simulink model "nuclearReactor"  (R2014b)
settings: Solver=ode1  StartTime=0.0  StopTime=100  FixedStep=0.0001  MaxStep=0.0001  RelTol=1e-3
(part 3 of 4)

== system nuclearReactor/Plant6 ==
  control : Inport
  Integrator t0 : DiscreteIntegrator  ExternalReset=either  InitialConditionSource=external  InitialCondition=510  InitialConditionSetting=State (most efficient)  SampleTime=-1
  Integrator t1 : DiscreteIntegrator  ExternalReset=either  InitialConditionSource=external  InitialCondition=510  InitialConditionSetting=State (most efficient)  SampleTime=-1
  Integrator t2 : DiscreteIntegrator  ExternalReset=either  InitialConditionSource=external  InitialCondition=510  InitialConditionSetting=State (most efficient)  SampleTime=-1
  MATLAB Function : MATLAB Function  Priority=1  TreatAsAtomicUnit=on
  MATLAB Function1 : MATLAB Function  Priority=1  TreatAsAtomicUnit=on
  Multiport Switch : MultiPortSwitch  DataPortOrder=Zero-based contiguous
  Scope : Scope  NumInputPorts=8
      settings: TickLabels=on  ShowLegends=on  YMin=0~0~0~10~1~1~0~-1  YMax=40~20~20~30~3~3~1~1
  THR3 : Constant  Value=510
  THR4 : Constant  Value=550
  THR5 : Constant  Value=550
  q : Memory  LinearizeMemory=on
  reset : Memory  LinearizeMemory=on
  x : Outport
  wires:
  Multiport Switch/1 -> Scope/1, MATLAB Function1/1(x), x/1  "x"
  MATLAB Function1/1(x_dot0) -> Integrator t0/1
  THR3/1 -> Integrator t0/3
  THR4/1 -> Integrator t1/3
  THR5/1 -> Integrator t2/3
  Integrator t0/1 -> Scope/2, Multiport Switch/2  "integrator t0"
  Integrator t1/1 -> Scope/3, Multiport Switch/3  "integrator t1"
  Integrator t2/1 -> Scope/4, Multiport Switch/4  "integrator t2"
  MATLAB Function1/2(x_dot1) -> Integrator t1/1
  MATLAB Function1/3(x_dot2) -> Integrator t2/1
  MATLAB Function/1(qNext) -> q/1  "q_before"
  q/1 -> MATLAB Function/1(q), Scope/5, Multiport Switch/1  "q_after"
  control/1 -> Scope/8, MATLAB Function/2(control)
  MATLAB Function/2(reset) -> reset/1
  reset/1 -> Integrator t0/2, Integrator t1/2, Integrator t2/2  "reset_after"

== system nuclearReactor/Plant7 ==
  control : Inport
  Integrator t0 : DiscreteIntegrator  ExternalReset=either  InitialConditionSource=external  InitialCondition=510  InitialConditionSetting=State (most efficient)  SampleTime=-1
  Integrator t1 : DiscreteIntegrator  ExternalReset=either  InitialConditionSource=external  InitialCondition=510  InitialConditionSetting=State (most efficient)  SampleTime=-1
  Integrator t2 : DiscreteIntegrator  ExternalReset=either  InitialConditionSource=external  InitialCondition=510  InitialConditionSetting=State (most efficient)  SampleTime=-1
  MATLAB Function : MATLAB Function  Priority=1  TreatAsAtomicUnit=on
  MATLAB Function1 : MATLAB Function  Priority=1  TreatAsAtomicUnit=on
  Multiport Switch : MultiPortSwitch  DataPortOrder=Zero-based contiguous
  Scope : Scope  NumInputPorts=8
      settings: TickLabels=on  ShowLegends=on  YMin=0~0~0~10~1~1~0~-1  YMax=40~20~20~30~3~3~1~1
  THR3 : Constant  Value=510
  THR4 : Constant  Value=550
  THR5 : Constant  Value=550
  q : Memory  LinearizeMemory=on
  reset : Memory  LinearizeMemory=on
  x : Outport
  wires:
  Multiport Switch/1 -> Scope/1, MATLAB Function1/1(x), x/1  "x"
  MATLAB Function1/1(x_dot0) -> Integrator t0/1
  THR3/1 -> Integrator t0/3
  THR4/1 -> Integrator t1/3
  THR5/1 -> Integrator t2/3
  Integrator t0/1 -> Scope/2, Multiport Switch/2  "integrator t0"
  Integrator t1/1 -> Scope/3, Multiport Switch/3  "integrator t1"
  Integrator t2/1 -> Scope/4, Multiport Switch/4  "integrator t2"
  MATLAB Function1/2(x_dot1) -> Integrator t1/1
  MATLAB Function1/3(x_dot2) -> Integrator t2/1
  MATLAB Function/1(qNext) -> q/1  "q_before"
  q/1 -> MATLAB Function/1(q), Scope/5, Multiport Switch/1  "q_after"
  control/1 -> Scope/8, MATLAB Function/2(control)
  MATLAB Function/2(reset) -> reset/1
  reset/1 -> Integrator t0/2, Integrator t1/2, Integrator t2/2  "reset_after"

== system nuclearReactor/Plant8 ==
  control : Inport
  Integrator t0 : DiscreteIntegrator  ExternalReset=either  InitialConditionSource=external  InitialCondition=510  InitialConditionSetting=State (most efficient)  SampleTime=-1
  Integrator t1 : DiscreteIntegrator  ExternalReset=either  InitialConditionSource=external  InitialCondition=510  InitialConditionSetting=State (most efficient)  SampleTime=-1
  Integrator t2 : DiscreteIntegrator  ExternalReset=either  InitialConditionSource=external  InitialCondition=510  InitialConditionSetting=State (most efficient)  SampleTime=-1
  MATLAB Function : MATLAB Function  Priority=1  TreatAsAtomicUnit=on
  MATLAB Function1 : MATLAB Function  Priority=1  TreatAsAtomicUnit=on
  Multiport Switch : MultiPortSwitch  DataPortOrder=Zero-based contiguous
  Scope : Scope  NumInputPorts=8
      settings: TickLabels=on  ShowLegends=on  YMin=0~0~0~10~1~1~0~-1  YMax=40~20~20~30~3~3~1~1
  THR3 : Constant  Value=510
  THR4 : Constant  Value=550
  THR5 : Constant  Value=550
  q : Memory  LinearizeMemory=on
  reset : Memory  LinearizeMemory=on
  x : Outport
  wires:
  Multiport Switch/1 -> Scope/1, MATLAB Function1/1(x), x/1  "x"
  MATLAB Function1/1(x_dot0) -> Integrator t0/1
  THR3/1 -> Integrator t0/3
  THR4/1 -> Integrator t1/3
  THR5/1 -> Integrator t2/3
  Integrator t0/1 -> Scope/2, Multiport Switch/2  "integrator t0"
  Integrator t1/1 -> Scope/3, Multiport Switch/3  "integrator t1"
  Integrator t2/1 -> Scope/4, Multiport Switch/4  "integrator t2"
  MATLAB Function1/2(x_dot1) -> Integrator t1/1
  MATLAB Function1/3(x_dot2) -> Integrator t2/1
  MATLAB Function/1(qNext) -> q/1  "q_before"
  q/1 -> MATLAB Function/1(q), Scope/5, Multiport Switch/1  "q_after"
  control/1 -> Scope/8, MATLAB Function/2(control)
  MATLAB Function/2(reset) -> reset/1
  reset/1 -> Integrator t0/2, Integrator t1/2, Integrator t2/2  "reset_after"

== system nuclearReactor/Plant9 ==
  control : Inport
  Integrator t0 : DiscreteIntegrator  ExternalReset=either  InitialConditionSource=external  InitialCondition=510  InitialConditionSetting=State (most efficient)  SampleTime=-1
  Integrator t1 : DiscreteIntegrator  ExternalReset=either  InitialConditionSource=external  InitialCondition=510  InitialConditionSetting=State (most efficient)  SampleTime=-1
  Integrator t2 : DiscreteIntegrator  ExternalReset=either  InitialConditionSource=external  InitialCondition=510  InitialConditionSetting=State (most efficient)  SampleTime=-1
  MATLAB Function : MATLAB Function  Priority=1  TreatAsAtomicUnit=on
  MATLAB Function1 : MATLAB Function  Priority=1  TreatAsAtomicUnit=on
  Multiport Switch : MultiPortSwitch  DataPortOrder=Zero-based contiguous
  Scope : Scope  NumInputPorts=8
      settings: TickLabels=on  ShowLegends=on  YMin=0~0~0~10~1~1~0~-1  YMax=40~20~20~30~3~3~1~1
  THR3 : Constant  Value=510
  THR4 : Constant  Value=550
  THR5 : Constant  Value=550
  q : Memory  LinearizeMemory=on
  reset : Memory  LinearizeMemory=on
  x : Outport
  wires:
  Multiport Switch/1 -> Scope/1, MATLAB Function1/1(x), x/1  "x"
  MATLAB Function1/1(x_dot0) -> Integrator t0/1
  THR3/1 -> Integrator t0/3
  THR4/1 -> Integrator t1/3
  THR5/1 -> Integrator t2/3
  Integrator t0/1 -> Scope/2, Multiport Switch/2  "integrator t0"
  Integrator t1/1 -> Scope/3, Multiport Switch/3  "integrator t1"
  Integrator t2/1 -> Scope/4, Multiport Switch/4  "integrator t2"
  MATLAB Function1/2(x_dot1) -> Integrator t1/1
  MATLAB Function1/3(x_dot2) -> Integrator t2/1
  MATLAB Function/1(qNext) -> q/1  "q_before"
  q/1 -> MATLAB Function/1(q), Scope/5, Multiport Switch/1  "q_after"
  control/1 -> Scope/8, MATLAB Function/2(control)
  MATLAB Function/2(reset) -> reset/1
  reset/1 -> Integrator t0/2, Integrator t1/2, Integrator t2/2  "reset_after"

== matlab function nuclearReactor/Plant/MATLAB Function ==
  data: q input; qNext output; control input; reset output


function [qNext,reset]  = phi(q, control)
%#codegen
% control {-1 undefined, 0 add1, 1 remove1, 2 add2, 3 remove2}

undef =0;
add1 = 1;
remove1 =2;
add2 = 3;
remove2 =4;
c=10;

if q==0 
    %When plant is in T0 ("No Rod")
    if control ==add1
        qNext=1;
        reset=1;
    elseif control ==add2
        qNext=2;
        reset=1;
    else
        qNext=0;
        reset=0;
    end;
    
elseif q==1    
    %When plant is in T1 ("Rod One")
    if control ==remove1
        qNext=0;
        reset=1;
    else
        qNext=1;
        reset=0;
    end;

elseif q==2    
    %When plant is in T2 ("Rod Two")
    if control ==remove2
        qNext=0;
        reset=1;
    else
        qNext=2;
        reset=0;
    end;
else
    qNext=-1; %this should never execute
    reset=-1; %this should never execute
end

== matlab function nuclearReactor/Controller/MATLAB Function ==
  data: q input; qNext output; x input; r1 output; r2 output; y1 input; y2 input; control output


function [qNext,r1,r2,control]  = phi(q, x, y1, y2)
%#codegen
% control {-1 undefined, 0 add1, 1 remove1, 2 add2, 3 remove2}

undef =0;
add1 = 1;
remove1 =2;
add2 = 3;
remove2 =4;
c=15;

if q==0 
    %When plant is in T0 ("No Rod")
    if x > 550 && y1 >= c && y2<c
        qNext=1;
        r1=0; r2=0;
        control=add1;
    elseif x>550 && y2>=c
        qNext=2;
        r1=0; r2=0;
        control=add2;
    else
        qNext=0;
        r1=0; r2=0;
        control=undef;
    end;
    
elseif q==1    
    %When plant is in T1 ("Rod One")
    if x <= 510 
        qNext=0;
        r1=1; r2=0;
        control=remove1;
    else
        qNext=1;
        r1=0; r2=0;
        control=undef;
    end;

elseif q==2    
    %When plant is in T2 ("Rod Two")
    if x <= 510 
        qNext=0;
        r1=0; r2=1;
        control=remove2;
    else
        qNext=2;
        r1=0; r2=0;
        control=undef;
    end;
else
    qNext=-1; %this should never execute
    r1=0; r2=0; %this should never execute
    control=-1; %this should never execute
end

== matlab function nuclearReactor/Plant/MATLAB Function1 ==
  data: x input; x_dot0 output; x_dot1 output; x_dot2 output
function [x_dot0, x_dot1, x_dot2] = ODEs(x)
%#codegen
x_dot0=0.1*x-50;
x_dot1=0.1*x-56;
x_dot2=0.1*x-60;

== matlab function nuclearReactor/Controller1/MATLAB Function ==
  data: q input; qNext output; x input; r1 output; r2 output; y1 input; y2 input; control output


function [qNext,r1,r2,control]  = phi(q, x, y1, y2)
%#codegen
% control {-1 undefined, 0 add1, 1 remove1, 2 add2, 3 remove2}

undef =0;
add1 = 1;
remove1 =2;
add2 = 3;
remove2 =4;
c=15;

if q==0 
    %When plant is in T0 ("No Rod")
    if x > 550 && y1 >= c && y2<c
        qNext=1;
        r1=0; r2=0;
        control=add1;
    elseif x>550 && y2>=c
        qNext=2;
        r1=0; r2=0;
        control=add2;
    else
        qNext=0;
        r1=0; r2=0;
        control=undef;
    end;
    
elseif q==1    
    %When plant is in T1 ("Rod One")
    if x <= 510 
        qNext=0;
        r1=1; r2=0;
        control=remove1;
    else
        qNext=1;
        r1=0; r2=0;
        control=undef;
    end;

elseif q==2    
    %When plant is in T2 ("Rod Two")
    if x <= 510 
        qNext=0;
        r1=0; r2=1;
        control=remove2;
    else
        qNext=2;
        r1=0; r2=0;
        control=undef;
    end;
else
    qNext=-1; %this should never execute
    r1=0; r2=0; %this should never execute
    control=-1; %this should never execute
end

== matlab function nuclearReactor/Plant1/MATLAB Function ==
  data: q input; qNext output; control input; reset output


function [qNext,reset]  = phi(q, control)
%#codegen
% control {-1 undefined, 0 add1, 1 remove1, 2 add2, 3 remove2}

undef =0;
add1 = 1;
remove1 =2;
add2 = 3;
remove2 =4;
c=10;

if q==0 
    %When plant is in T0 ("No Rod")
    if control ==add1
        qNext=1;
        reset=1;
    elseif control ==add2
        qNext=2;
        reset=1;
    else
        qNext=0;
        reset=0;
    end;
    
elseif q==1    
    %When plant is in T1 ("Rod One")
    if control ==remove1
        qNext=0;
        reset=1;
    else
        qNext=1;
        reset=0;
    end;

elseif q==2    
    %When plant is in T2 ("Rod Two")
    if control ==remove2
        qNext=0;
        reset=1;
    else
        qNext=2;
        reset=0;
    end;
else
    qNext=-1; %this should never execute
    reset=-1; %this should never execute
end

== matlab function nuclearReactor/Plant1/MATLAB Function1 ==
  data: x input; x_dot0 output; x_dot1 output; x_dot2 output
function [x_dot0, x_dot1, x_dot2] = ODEs(x)
%#codegen
x_dot0=0.1*x-50;
x_dot1=0.1*x-56;
x_dot2=0.1*x-60;

== matlab function nuclearReactor/Controller2/MATLAB Function ==
  data: q input; qNext output; x input; r1 output; r2 output; y1 input; y2 input; control output


function [qNext,r1,r2,control]  = phi(q, x, y1, y2)
%#codegen
% control {-1 undefined, 0 add1, 1 remove1, 2 add2, 3 remove2}

undef =0;
add1 = 1;
remove1 =2;
add2 = 3;
remove2 =4;
c=15;

if q==0 
    %When plant is in T0 ("No Rod")
    if x > 550 && y1 >= c && y2<c
        qNext=1;
        r1=0; r2=0;
        control=add1;
    elseif x>550 && y2>=c
        qNext=2;
        r1=0; r2=0;
        control=add2;
    else
        qNext=0;
        r1=0; r2=0;
        control=undef;
    end;
    
elseif q==1    
    %When plant is in T1 ("Rod One")
    if x <= 510 
        qNext=0;
        r1=1; r2=0;
        control=remove1;
    else
        qNext=1;
        r1=0; r2=0;
        control=undef;
    end;

elseif q==2    
    %When plant is in T2 ("Rod Two")
    if x <= 510 
        qNext=0;
        r1=0; r2=1;
        control=remove2;
    else
        qNext=2;
        r1=0; r2=0;
        control=undef;
    end;
else
    qNext=-1; %this should never execute
    r1=0; r2=0; %this should never execute
    control=-1; %this should never execute
end

== matlab function nuclearReactor/Plant2/MATLAB Function ==
  data: q input; qNext output; control input; reset output


function [qNext,reset]  = phi(q, control)
%#codegen
% control {-1 undefined, 0 add1, 1 remove1, 2 add2, 3 remove2}

undef =0;
add1 = 1;
remove1 =2;
add2 = 3;
remove2 =4;
c=10;

if q==0 
    %When plant is in T0 ("No Rod")
    if control ==add1
        qNext=1;
        reset=1;
    elseif control ==add2
        qNext=2;
        reset=1;
    else
        qNext=0;
        reset=0;
    end;
    
elseif q==1    
    %When plant is in T1 ("Rod One")
    if control ==remove1
        qNext=0;
        reset=1;
    else
        qNext=1;
        reset=0;
    end;

elseif q==2    
    %When plant is in T2 ("Rod Two")
    if control ==remove2
        qNext=0;
        reset=1;
    else
        qNext=2;
        reset=0;
    end;
else
    qNext=-1; %this should never execute
    reset=-1; %this should never execute
end

== matlab function nuclearReactor/Plant2/MATLAB Function1 ==
  data: x input; x_dot0 output; x_dot1 output; x_dot2 output
function [x_dot0, x_dot1, x_dot2] = ODEs(x)
%#codegen
x_dot0=0.1*x-50;
x_dot1=0.1*x-56;
x_dot2=0.1*x-60;

== matlab function nuclearReactor/Controller3/MATLAB Function ==
  data: q input; qNext output; x input; r1 output; r2 output; y1 input; y2 input; control output


function [qNext,r1,r2,control]  = phi(q, x, y1, y2)
%#codegen
% control {-1 undefined, 0 add1, 1 remove1, 2 add2, 3 remove2}

undef =0;
add1 = 1;
remove1 =2;
add2 = 3;
remove2 =4;
c=15;

if q==0 
    %When plant is in T0 ("No Rod")
    if x > 550 && y1 >= c && y2<c
        qNext=1;
        r1=0; r2=0;
        control=add1;
    elseif x>550 && y2>=c
        qNext=2;
        r1=0; r2=0;
        control=add2;
    else
        qNext=0;
        r1=0; r2=0;
        control=undef;
    end;
    
elseif q==1    
    %When plant is in T1 ("Rod One")
    if x <= 510 
        qNext=0;
        r1=1; r2=0;
        control=remove1;
    else
        qNext=1;
        r1=0; r2=0;
        control=undef;
    end;

elseif q==2    
    %When plant is in T2 ("Rod Two")
    if x <= 510 
        qNext=0;
        r1=0; r2=1;
        control=remove2;
    else
        qNext=2;
        r1=0; r2=0;
        control=undef;
    end;
else
    qNext=-1; %this should never execute
    r1=0; r2=0; %this should never execute
    control=-1; %this should never execute
end

== matlab function nuclearReactor/Plant3/MATLAB Function ==
  data: q input; qNext output; control input; reset output


function [qNext,reset]  = phi(q, control)
%#codegen
% control {-1 undefined, 0 add1, 1 remove1, 2 add2, 3 remove2}

undef =0;
add1 = 1;
remove1 =2;
add2 = 3;
remove2 =4;
c=10;

if q==0 
    %When plant is in T0 ("No Rod")
    if control ==add1
        qNext=1;
        reset=1;
    elseif control ==add2
        qNext=2;
        reset=1;
    else
        qNext=0;
        reset=0;
    end;
    
elseif q==1    
    %When plant is in T1 ("Rod One")
    if control ==remove1
        qNext=0;
        reset=1;
    else
        qNext=1;
        reset=0;
    end;

elseif q==2    
    %When plant is in T2 ("Rod Two")
    if control ==remove2
        qNext=0;
        reset=1;
    else
        qNext=2;
        reset=0;
    end;
else
    qNext=-1; %this should never execute
    reset=-1; %this should never execute
end

== matlab function nuclearReactor/Plant3/MATLAB Function1 ==
  data: x input; x_dot0 output; x_dot1 output; x_dot2 output
function [x_dot0, x_dot1, x_dot2] = ODEs(x)
%#codegen
x_dot0=0.1*x-50;
x_dot1=0.1*x-56;
x_dot2=0.1*x-60;

== matlab function nuclearReactor/Controller4/MATLAB Function ==
  data: q input; qNext output; x input; r1 output; r2 output; y1 input; y2 input; control output


function [qNext,r1,r2,control]  = phi(q, x, y1, y2)
%#codegen
% control {-1 undefined, 0 add1, 1 remove1, 2 add2, 3 remove2}

undef =0;
add1 = 1;
remove1 =2;
add2 = 3;
remove2 =4;
c=15;

if q==0 
    %When plant is in T0 ("No Rod")
    if x > 550 && y1 >= c && y2<c
        qNext=1;
        r1=0; r2=0;
        control=add1;
    elseif x>550 && y2>=c
        qNext=2;
        r1=0; r2=0;
        control=add2;
    else
        qNext=0;
        r1=0; r2=0;
        control=undef;
    end;
    
elseif q==1    
    %When plant is in T1 ("Rod One")
    if x <= 510 
        qNext=0;
        r1=1; r2=0;
        control=remove1;
    else
        qNext=1;
        r1=0; r2=0;
        control=undef;
    end;

elseif q==2    
    %When plant is in T2 ("Rod Two")
    if x <= 510 
        qNext=0;
        r1=0; r2=1;
        control=remove2;
    else
        qNext=2;
        r1=0; r2=0;
        control=undef;
    end;
else
    qNext=-1; %this should never execute
    r1=0; r2=0; %this should never execute
    control=-1; %this should never execute
end

== matlab function nuclearReactor/Plant4/MATLAB Function ==
  data: q input; qNext output; control input; reset output


function [qNext,reset]  = phi(q, control)
%#codegen
% control {-1 undefined, 0 add1, 1 remove1, 2 add2, 3 remove2}

undef =0;
add1 = 1;
remove1 =2;
add2 = 3;
remove2 =4;
c=10;

if q==0 
    %When plant is in T0 ("No Rod")
    if control ==add1
        qNext=1;
        reset=1;
    elseif control ==add2
        qNext=2;
        reset=1;
    else
        qNext=0;
        reset=0;
    end;
    
elseif q==1    
    %When plant is in T1 ("Rod One")
    if control ==remove1
        qNext=0;
        reset=1;
    else
        qNext=1;
        reset=0;
    end;

elseif q==2    
    %When plant is in T2 ("Rod Two")
    if control ==remove2
        qNext=0;
        reset=1;
    else
        qNext=2;
        reset=0;
    end;
else
    qNext=-1; %this should never execute
    reset=-1; %this should never execute
end

== matlab function nuclearReactor/Plant4/MATLAB Function1 ==
  data: x input; x_dot0 output; x_dot1 output; x_dot2 output
function [x_dot0, x_dot1, x_dot2] = ODEs(x)
%#codegen
x_dot0=0.1*x-50;
x_dot1=0.1*x-56;
x_dot2=0.1*x-60;

== matlab function nuclearReactor/Controller5/MATLAB Function ==
  data: q input; qNext output; x input; r1 output; r2 output; y1 input; y2 input; control output


function [qNext,r1,r2,control]  = phi(q, x, y1, y2)
%#codegen
% control {-1 undefined, 0 add1, 1 remove1, 2 add2, 3 remove2}

undef =0;
add1 = 1;
remove1 =2;
add2 = 3;
remove2 =4;
c=15;

if q==0 
    %When plant is in T0 ("No Rod")
    if x > 550 && y1 >= c && y2<c
        qNext=1;
        r1=0; r2=0;
        control=add1;
    elseif x>550 && y2>=c
        qNext=2;
        r1=0; r2=0;
        control=add2;
    else
        qNext=0;
        r1=0; r2=0;
        control=undef;
    end;
    
elseif q==1    
    %When plant is in T1 ("Rod One")
    if x <= 510 
        qNext=0;
        r1=1; r2=0;
        control=remove1;
    else
        qNext=1;
        r1=0; r2=0;
        control=undef;
    end;

elseif q==2    
    %When plant is in T2 ("Rod Two")
    if x <= 510 
        qNext=0;
        r1=0; r2=1;
        control=remove2;
    else
        qNext=2;
        r1=0; r2=0;
        control=undef;
    end;
else
    qNext=-1; %this should never execute
    r1=0; r2=0; %this should never execute
    control=-1; %this should never execute
end

== matlab function nuclearReactor/Plant5/MATLAB Function ==
  data: q input; qNext output; control input; reset output


function [qNext,reset]  = phi(q, control)
%#codegen
% control {-1 undefined, 0 add1, 1 remove1, 2 add2, 3 remove2}

undef =0;
add1 = 1;
remove1 =2;
add2 = 3;
remove2 =4;
c=10;

if q==0 
    %When plant is in T0 ("No Rod")
    if control ==add1
        qNext=1;
        reset=1;
    elseif control ==add2
        qNext=2;
        reset=1;
    else
        qNext=0;
        reset=0;
    end;
    
elseif q==1    
    %When plant is in T1 ("Rod One")
    if control ==remove1
        qNext=0;
        reset=1;
    else
        qNext=1;
        reset=0;
    end;

elseif q==2    
    %When plant is in T2 ("Rod Two")
    if control ==remove2
        qNext=0;
        reset=1;
    else
        qNext=2;
        reset=0;
    end;
else
    qNext=-1; %this should never execute
    reset=-1; %this should never execute
end

== matlab function nuclearReactor/Plant5/MATLAB Function1 ==
  data: x input; x_dot0 output; x_dot1 output; x_dot2 output
function [x_dot0, x_dot1, x_dot2] = ODEs(x)
%#codegen
x_dot0=0.1*x-50;
x_dot1=0.1*x-56;
x_dot2=0.1*x-60;

== matlab function nuclearReactor/Controller6/MATLAB Function ==
  data: q input; qNext output; x input; r1 output; r2 output; y1 input; y2 input; control output


function [qNext,r1,r2,control]  = phi(q, x, y1, y2)
%#codegen
% control {-1 undefined, 0 add1, 1 remove1, 2 add2, 3 remove2}

undef =0;
add1 = 1;
remove1 =2;
add2 = 3;
remove2 =4;
c=15;

if q==0 
    %When plant is in T0 ("No Rod")
    if x > 550 && y1 >= c && y2<c
        qNext=1;
        r1=0; r2=0;
        control=add1;
    elseif x>550 && y2>=c
        qNext=2;
        r1=0; r2=0;
        control=add2;
    else
        qNext=0;
        r1=0; r2=0;
        control=undef;
    end;
    
elseif q==1    
    %When plant is in T1 ("Rod One")
    if x <= 510 
        qNext=0;
        r1=1; r2=0;
        control=remove1;
    else
        qNext=1;
        r1=0; r2=0;
        control=undef;
    end;

elseif q==2    
    %When plant is in T2 ("Rod Two")
    if x <= 510 
        qNext=0;
        r1=0; r2=1;
        control=remove2;
    else
        qNext=2;
        r1=0; r2=0;
        control=undef;
    end;
else
    qNext=-1; %this should never execute
    r1=0; r2=0; %this should never execute
    control=-1; %this should never execute
end

== matlab function nuclearReactor/Plant6/MATLAB Function ==
  data: q input; qNext output; control input; reset output


function [qNext,reset]  = phi(q, control)
%#codegen
% control {-1 undefined, 0 add1, 1 remove1, 2 add2, 3 remove2}

undef =0;
add1 = 1;
remove1 =2;
add2 = 3;
remove2 =4;
c=10;

if q==0 
    %When plant is in T0 ("No Rod")
    if control ==add1
        qNext=1;
        reset=1;
    elseif control ==add2
        qNext=2;
        reset=1;
    else
        qNext=0;
        reset=0;
    end;
    
elseif q==1    
    %When plant is in T1 ("Rod One")
    if control ==remove1
        qNext=0;
        reset=1;
    else
        qNext=1;
        reset=0;
    end;

elseif q==2    
    %When plant is in T2 ("Rod Two")
    if control ==remove2
        qNext=0;
        reset=1;
    else
        qNext=2;
        reset=0;
    end;
else
    qNext=-1; %this should never execute
    reset=-1; %this should never execute
end

== matlab function nuclearReactor/Plant6/MATLAB Function1 ==
  data: x input; x_dot0 output; x_dot1 output; x_dot2 output
function [x_dot0, x_dot1, x_dot2] = ODEs(x)
%#codegen
x_dot0=0.1*x-50;
x_dot1=0.1*x-56;
x_dot2=0.1*x-60;

== matlab function nuclearReactor/Controller7/MATLAB Function ==
  data: q input; qNext output; x input; r1 output; r2 output; y1 input; y2 input; control output


function [qNext,r1,r2,control]  = phi(q, x, y1, y2)
%#codegen
% control {-1 undefined, 0 add1, 1 remove1, 2 add2, 3 remove2}

undef =0;
add1 = 1;
remove1 =2;
add2 = 3;
remove2 =4;
c=15;

if q==0 
    %When plant is in T0 ("No Rod")
    if x > 550 && y1 >= c && y2<c
        qNext=1;
        r1=0; r2=0;
        control=add1;
    elseif x>550 && y2>=c
        qNext=2;
        r1=0; r2=0;
        control=add2;
    else
        qNext=0;
        r1=0; r2=0;
        control=undef;
    end;
    
elseif q==1    
    %When plant is in T1 ("Rod One")
    if x <= 510 
        qNext=0;
        r1=1; r2=0;
        control=remove1;
    else
        qNext=1;
        r1=0; r2=0;
        control=undef;
    end;

elseif q==2    
    %When plant is in T2 ("Rod Two")
    if x <= 510 
        qNext=0;
        r1=0; r2=1;
        control=remove2;
    else
        qNext=2;
        r1=0; r2=0;
        control=undef;
    end;
else
    qNext=-1; %this should never execute
    r1=0; r2=0; %this should never execute
    control=-1; %this should never execute
end

== matlab function nuclearReactor/Plant7/MATLAB Function ==
  data: q input; qNext output; control input; reset output


function [qNext,reset]  = phi(q, control)
%#codegen
% control {-1 undefined, 0 add1, 1 remove1, 2 add2, 3 remove2}

undef =0;
add1 = 1;
remove1 =2;
add2 = 3;
remove2 =4;
c=10;

if q==0 
    %When plant is in T0 ("No Rod")
    if control ==add1
        qNext=1;
        reset=1;
    elseif control ==add2
        qNext=2;
        reset=1;
    else
        qNext=0;
        reset=0;
    end;
    
elseif q==1    
    %When plant is in T1 ("Rod One")
    if control ==remove1
        qNext=0;
        reset=1;
    else
        qNext=1;
        reset=0;
    end;

elseif q==2    
    %When plant is in T2 ("Rod Two")
    if control ==remove2
        qNext=0;
        reset=1;
    else
        qNext=2;
        reset=0;
    end;
else
    qNext=-1; %this should never execute
    reset=-1; %this should never execute
end

== matlab function nuclearReactor/Plant7/MATLAB Function1 ==
  data: x input; x_dot0 output; x_dot1 output; x_dot2 output
function [x_dot0, x_dot1, x_dot2] = ODEs(x)
%#codegen
x_dot0=0.1*x-50;
x_dot1=0.1*x-56;
x_dot2=0.1*x-60;

== matlab function nuclearReactor/Controller8/MATLAB Function ==
  data: q input; qNext output; x input; r1 output; r2 output; y1 input; y2 input; control output


function [qNext,r1,r2,control]  = phi(q, x, y1, y2)
%#codegen
% control {-1 undefined, 0 add1, 1 remove1, 2 add2, 3 remove2}

undef =0;
add1 = 1;
remove1 =2;
add2 = 3;
remove2 =4;
c=15;

if q==0 
    %When plant is in T0 ("No Rod")
    if x > 550 && y1 >= c && y2<c
        qNext=1;
        r1=0; r2=0;
        control=add1;
    elseif x>550 && y2>=c
        qNext=2;
        r1=0; r2=0;
        control=add2;
    else
        qNext=0;
        r1=0; r2=0;
        control=undef;
    end;
    
elseif q==1    
    %When plant is in T1 ("Rod One")
    if x <= 510 
        qNext=0;
        r1=1; r2=0;
        control=remove1;
    else
        qNext=1;
        r1=0; r2=0;
        control=undef;
    end;

elseif q==2    
    %When plant is in T2 ("Rod Two")
    if x <= 510 
        qNext=0;
        r1=0; r2=1;
        control=remove2;
    else
        qNext=2;
        r1=0; r2=0;
        control=undef;
    end;
else
    qNext=-1; %this should never execute
    r1=0; r2=0; %this should never execute
    control=-1; %this should never execute
end

== matlab function nuclearReactor/Plant8/MATLAB Function ==
  data: q input; qNext output; control input; reset output


function [qNext,reset]  = phi(q, control)
%#codegen
% control {-1 undefined, 0 add1, 1 remove1, 2 add2, 3 remove2}

undef =0;
add1 = 1;
remove1 =2;
add2 = 3;
remove2 =4;
c=10;

if q==0 
    %When plant is in T0 ("No Rod")
    if control ==add1
        qNext=1;
        reset=1;
    elseif control ==add2
        qNext=2;
        reset=1;
    else
        qNext=0;
        reset=0;
    end;
    
elseif q==1    
    %When plant is in T1 ("Rod One")
    if control ==remove1
        qNext=0;
        reset=1;
    else
        qNext=1;
        reset=0;
    end;

elseif q==2    
    %When plant is in T2 ("Rod Two")
    if control ==remove2
        qNext=0;
        reset=1;
    else
        qNext=2;
        reset=0;
    end;
else
    qNext=-1; %this should never execute
    reset=-1; %this should never execute
end

== matlab function nuclearReactor/Plant8/MATLAB Function1 ==
  data: x input; x_dot0 output; x_dot1 output; x_dot2 output
function [x_dot0, x_dot1, x_dot2] = ODEs(x)
%#codegen
x_dot0=0.1*x-50;
x_dot1=0.1*x-56;
x_dot2=0.1*x-60;

== matlab function nuclearReactor/Controller9/MATLAB Function ==
  data: q input; qNext output; x input; r1 output; r2 output; y1 input; y2 input; control output


function [qNext,r1,r2,control]  = phi(q, x, y1, y2)
%#codegen
% control {-1 undefined, 0 add1, 1 remove1, 2 add2, 3 remove2}

undef =0;
add1 = 1;
remove1 =2;
add2 = 3;
remove2 =4;
c=15;

if q==0 
    %When plant is in T0 ("No Rod")
    if x > 550 && y1 >= c && y2<c
        qNext=1;
        r1=0; r2=0;
        control=add1;
    elseif x>550 && y2>=c
        qNext=2;
        r1=0; r2=0;
        control=add2;
    else
        qNext=0;
        r1=0; r2=0;
        control=undef;
    end;
    
elseif q==1    
    %When plant is in T1 ("Rod One")
    if x <= 510 
        qNext=0;
        r1=1; r2=0;
        control=remove1;
    else
        qNext=1;
        r1=0; r2=0;
        control=undef;
    end;

elseif q==2    
    %When plant is in T2 ("Rod Two")
    if x <= 510 
        qNext=0;
        r1=0; r2=1;
        control=remove2;
    else
        qNext=2;
        r1=0; r2=0;
        control=undef;
    end;
else
    qNext=-1; %this should never execute
    r1=0; r2=0; %this should never execute
    control=-1; %this should never execute
end

== matlab function nuclearReactor/Plant9/MATLAB Function ==
  data: q input; qNext output; control input; reset output


function [qNext,reset]  = phi(q, control)
%#codegen
% control {-1 undefined, 0 add1, 1 remove1, 2 add2, 3 remove2}

undef =0;
add1 = 1;
remove1 =2;
add2 = 3;
remove2 =4;
c=10;

if q==0 
    %When plant is in T0 ("No Rod")
    if control ==add1
        qNext=1;
        reset=1;
    elseif control ==add2
        qNext=2;
        reset=1;
    else
        qNext=0;
        reset=0;
    end;
    
elseif q==1    
    %When plant is in T1 ("Rod One")
    if control ==remove1
        qNext=0;
        reset=1;
    else
        qNext=1;
        reset=0;
    end;

elseif q==2    
    %When plant is in T2 ("Rod Two")
    if control ==remove2
        qNext=0;
        reset=1;
    else
        qNext=2;
        reset=0;
    end;
else
    qNext=-1; %this should never execute
    reset=-1; %this should never execute
end

== matlab function nuclearReactor/Plant9/MATLAB Function1 ==
  data: x input; x_dot0 output; x_dot1 output; x_dot2 output
function [x_dot0, x_dot1, x_dot2] = ODEs(x)
%#codegen
x_dot0=0.1*x-50;
x_dot1=0.1*x-56;
x_dot2=0.1*x-60;

== matlab function nuclearReactor/Controller10/MATLAB Function ==
  data: q input; qNext output; x input; r1 output; r2 output; y1 input; y2 input; control output


function [qNext,r1,r2,control]  = phi(q, x, y1, y2)
%#codegen
% control {-1 undefined, 0 add1, 1 remove1, 2 add2, 3 remove2}

undef =0;
add1 = 1;
remove1 =2;
add2 = 3;
remove2 =4;
c=15;

if q==0 
    %When plant is in T0 ("No Rod")
    if x > 550 && y1 >= c && y2<c
        qNext=1;
        r1=0; r2=0;
        control=add1;
    elseif x>550 && y2>=c
        qNext=2;
        r1=0; r2=0;
        control=add2;
    else
        qNext=0;
        r1=0; r2=0;
        control=undef;
    end;
    
elseif q==1    
    %When plant is in T1 ("Rod One")
    if x <= 510 
        qNext=0;
        r1=1; r2=0;
        control=remove1;
    else
        qNext=1;
        r1=0; r2=0;
        control=undef;
    end;

elseif q==2    
    %When plant is in T2 ("Rod Two")
    if x <= 510 
        qNext=0;
        r1=0; r2=1;
        control=remove2;
    else
        qNext=2;
        r1=0; r2=0;
        control=undef;
    end;
else
    qNext=-1; %this should never execute
    r1=0; r2=0; %this should never execute
    control=-1; %this should never execute
end

== matlab function nuclearReactor/Plant10/MATLAB Function ==
  data: q input; qNext output; control input; reset output


function [qNext,reset]  = phi(q, control)
%#codegen
% control {-1 undefined, 0 add1, 1 remove1, 2 add2, 3 remove2}

undef =0;
add1 = 1;
remove1 =2;
add2 = 3;
remove2 =4;
c=10;

if q==0 
    %When plant is in T0 ("No Rod")
    if control ==add1
        qNext=1;
        reset=1;
    elseif control ==add2
        qNext=2;
        reset=1;
    else
        qNext=0;
        reset=0;
    end;
    
elseif q==1    
    %When plant is in T1 ("Rod One")
    if control ==remove1
        qNext=0;
        reset=1;
    else
        qNext=1;
        reset=0;
    end;

elseif q==2    
    %When plant is in T2 ("Rod Two")
    if control ==remove2
        qNext=0;
        reset=1;
    else
        qNext=2;
        reset=0;
    end;
else
    qNext=-1; %this should never execute
    reset=-1; %this should never execute
end

== matlab function nuclearReactor/Plant10/MATLAB Function1 ==
  data: x input; x_dot0 output; x_dot1 output; x_dot2 output
function [x_dot0, x_dot1, x_dot2] = ODEs(x)
%#codegen
x_dot0=0.1*x-50;
x_dot1=0.1*x-56;
x_dot2=0.1*x-60;

== matlab function nuclearReactor/Controller11/MATLAB Function ==
  data: q input; qNext output; x input; r1 output; r2 output; y1 input; y2 input; control output


function [qNext,r1,r2,control]  = phi(q, x, y1, y2)
%#codegen
% control {-1 undefined, 0 add1, 1 remove1, 2 add2, 3 remove2}

undef =0;
add1 = 1;
remove1 =2;
add2 = 3;
remove2 =4;
c=15;

if q==0 
    %When plant is in T0 ("No Rod")
    if x > 550 && y1 >= c && y2<c
        qNext=1;
        r1=0; r2=0;
        control=add1;
    elseif x>550 && y2>=c
        qNext=2;
        r1=0; r2=0;
        control=add2;
    else
        qNext=0;
        r1=0; r2=0;
        control=undef;
    end;
    
elseif q==1    
    %When plant is in T1 ("Rod One")
    if x <= 510 
        qNext=0;
        r1=1; r2=0;
        control=remove1;
    else
        qNext=1;
        r1=0; r2=0;
        control=undef;
    end;

elseif q==2    
    %When plant is in T2 ("Rod Two")
    if x <= 510 
        qNext=0;
        r1=0; r2=1;
        control=remove2;
    else
        qNext=2;
        r1=0; r2=0;
        control=undef;
    end;
else
    qNext=-1; %this should never execute
    r1=0; r2=0; %this should never execute
    control=-1; %this should never execute
end

== matlab function nuclearReactor/Plant11/MATLAB Function ==
  data: q input; qNext output; control input; reset output


function [qNext,reset]  = phi(q, control)
%#codegen
% control {-1 undefined, 0 add1, 1 remove1, 2 add2, 3 remove2}

undef =0;
add1 = 1;
remove1 =2;
add2 = 3;
remove2 =4;
c=10;

if q==0 
    %When plant is in T0 ("No Rod")
    if control ==add1
        qNext=1;
        reset=1;
    elseif control ==add2
        qNext=2;
        reset=1;
    else
        qNext=0;
        reset=0;
    end;
    
elseif q==1    
    %When plant is in T1 ("Rod One")
    if control ==remove1
        qNext=0;
        reset=1;
    else
        qNext=1;
        reset=0;
    end;

elseif q==2    
    %When plant is in T2 ("Rod Two")
    if control ==remove2
        qNext=0;
        reset=1;
    else
        qNext=2;
        reset=0;
    end;
else
    qNext=-1; %this should never execute
    reset=-1; %this should never execute
end

== matlab function nuclearReactor/Plant11/MATLAB Function1 ==
  data: x input; x_dot0 output; x_dot1 output; x_dot2 output
function [x_dot0, x_dot1, x_dot2] = ODEs(x)
%#codegen
x_dot0=0.1*x-50;
x_dot1=0.1*x-56;
x_dot2=0.1*x-60;

== matlab function nuclearReactor/Controller12/MATLAB Function ==
  data: q input; qNext output; x input; r1 output; r2 output; y1 input; y2 input; control output


function [qNext,r1,r2,control]  = phi(q, x, y1, y2)
%#codegen
% control {-1 undefined, 0 add1, 1 remove1, 2 add2, 3 remove2}

undef =0;
add1 = 1;
remove1 =2;
add2 = 3;
remove2 =4;
c=15;

if q==0 
    %When plant is in T0 ("No Rod")
    if x > 550 && y1 >= c && y2<c
        qNext=1;
        r1=0; r2=0;
        control=add1;
    elseif x>550 && y2>=c
        qNext=2;
        r1=0; r2=0;
        control=add2;
    else
        qNext=0;
        r1=0; r2=0;
        control=undef;
    end;
    
elseif q==1    
    %When plant is in T1 ("Rod One")
    if x <= 510 
        qNext=0;
        r1=1; r2=0;
        control=remove1;
    else
        qNext=1;
        r1=0; r2=0;
        control=undef;
    end;

elseif q==2    
    %When plant is in T2 ("Rod Two")
    if x <= 510 
        qNext=0;
        r1=0; r2=1;
        control=remove2;
    else
        qNext=2;
        r1=0; r2=0;
        control=undef;
    end;
else
    qNext=-1; %this should never execute
    r1=0; r2=0; %this should never execute
    control=-1; %this should never execute
end

== matlab function nuclearReactor/Plant12/MATLAB Function ==
  data: q input; qNext output; control input; reset output


function [qNext,reset]  = phi(q, control)
%#codegen
% control {-1 undefined, 0 add1, 1 remove1, 2 add2, 3 remove2}

undef =0;
add1 = 1;
remove1 =2;
add2 = 3;
remove2 =4;
c=10;

if q==0 
    %When plant is in T0 ("No Rod")
    if control ==add1
        qNext=1;
        reset=1;
    elseif control ==add2
        qNext=2;
        reset=1;
    else
        qNext=0;
        reset=0;
    end;
    
elseif q==1    
    %When plant is in T1 ("Rod One")
    if control ==remove1
        qNext=0;
        reset=1;
    else
        qNext=1;
        reset=0;
    end;

elseif q==2    
    %When plant is in T2 ("Rod Two")
    if control ==remove2
        qNext=0;
        reset=1;
    else
        qNext=2;
        reset=0;
    end;
else
    qNext=-1; %this should never execute
    reset=-1; %this should never execute
end

== matlab function nuclearReactor/Plant12/MATLAB Function1 ==
  data: x input; x_dot0 output; x_dot1 output; x_dot2 output
function [x_dot0, x_dot1, x_dot2] = ODEs(x)
%#codegen
x_dot0=0.1*x-50;
x_dot1=0.1*x-56;
x_dot2=0.1*x-60;

== matlab function nuclearReactor/Controller13/MATLAB Function ==
  data: q input; qNext output; x input; r1 output; r2 output; y1 input; y2 input; control output


function [qNext,r1,r2,control]  = phi(q, x, y1, y2)
%#codegen
% control {-1 undefined, 0 add1, 1 remove1, 2 add2, 3 remove2}

undef =0;
add1 = 1;
remove1 =2;
add2 = 3;
remove2 =4;
c=15;

if q==0 
    %When plant is in T0 ("No Rod")
    if x > 550 && y1 >= c && y2<c
        qNext=1;
        r1=0; r2=0;
        control=add1;
    elseif x>550 && y2>=c
        qNext=2;
        r1=0; r2=0;
        control=add2;
    else
        qNext=0;
        r1=0; r2=0;
        control=undef;
    end;
    
elseif q==1    
    %When plant is in T1 ("Rod One")
    if x <= 510 
        qNext=0;
        r1=1; r2=0;
        control=remove1;
    else
        qNext=1;
        r1=0; r2=0;
        control=undef;
    end;

elseif q==2    
    %When plant is in T2 ("Rod Two")
    if x <= 510 
        qNext=0;
        r1=0; r2=1;
        control=remove2;
    else
        qNext=2;
        r1=0; r2=0;
        control=undef;
    end;
else
    qNext=-1; %this should never execute
    r1=0; r2=0; %this should never execute
    control=-1; %this should never execute
end

== matlab function nuclearReactor/Plant13/MATLAB Function ==
  data: q input; qNext output; control input; reset output


function [qNext,reset]  = phi(q, control)
%#codegen
% control {-1 undefined, 0 add1, 1 remove1, 2 add2, 3 remove2}

undef =0;
add1 = 1;
remove1 =2;
add2 = 3;
remove2 =4;
c=10;

if q==0 
    %When plant is in T0 ("No Rod")
    if control ==add1
        qNext=1;
        reset=1;
    elseif control ==add2
        qNext=2;
        reset=1;
    else
        qNext=0;
        reset=0;
    end;
    
elseif q==1    
    %When plant is in T1 ("Rod One")
    if control ==remove1
        qNext=0;
        reset=1;
    else
        qNext=1;
        reset=0;
    end;

elseif q==2    
    %When plant is in T2 ("Rod Two")
    if control ==remove2
        qNext=0;
        reset=1;
    else
        qNext=2;
        reset=0;
    end;
else
    qNext=-1; %this should never execute
    reset=-1; %this should never execute
end

== matlab function nuclearReactor/Plant13/MATLAB Function1 ==
  data: x input; x_dot0 output; x_dot1 output; x_dot2 output
function [x_dot0, x_dot1, x_dot2] = ODEs(x)
%#codegen
x_dot0=0.1*x-50;
x_dot1=0.1*x-56;
x_dot2=0.1*x-60;

== matlab function nuclearReactor/Controller14/MATLAB Function ==
  data: q input; qNext output; x input; r1 output; r2 output; y1 input; y2 input; control output


function [qNext,r1,r2,control]  = phi(q, x, y1, y2)
%#codegen
% control {-1 undefined, 0 add1, 1 remove1, 2 add2, 3 remove2}

undef =0;
add1 = 1;
remove1 =2;
add2 = 3;
remove2 =4;
c=15;

if q==0 
    %When plant is in T0 ("No Rod")
    if x > 550 && y1 >= c && y2<c
        qNext=1;
        r1=0; r2=0;
        control=add1;
    elseif x>550 && y2>=c
        qNext=2;
        r1=0; r2=0;
        control=add2;
    else
        qNext=0;
        r1=0; r2=0;
        control=undef;
    end;
    
elseif q==1    
    %When plant is in T1 ("Rod One")
    if x <= 510 
        qNext=0;
        r1=1; r2=0;
        control=remove1;
    else
        qNext=1;
        r1=0; r2=0;
        control=undef;
    end;

elseif q==2    
    %When plant is in T2 ("Rod Two")
    if x <= 510 
        qNext=0;
        r1=0; r2=1;
        control=remove2;
    else
        qNext=2;
        r1=0; r2=0;
        control=undef;
    end;
else
    qNext=-1; %this should never execute
    r1=0; r2=0; %this should never execute
    control=-1; %this should never execute
end

== matlab function nuclearReactor/Plant14/MATLAB Function ==
  data: q input; qNext output; control input; reset output


function [qNext,reset]  = phi(q, control)
%#codegen
% control {-1 undefined, 0 add1, 1 remove1, 2 add2, 3 remove2}

undef =0;
add1 = 1;
remove1 =2;
add2 = 3;
remove2 =4;
c=10;

if q==0 
    %When plant is in T0 ("No Rod")
    if control ==add1
        qNext=1;
        reset=1;
    elseif control ==add2
        qNext=2;
        reset=1;
    else
        qNext=0;
        reset=0;
    end;
    
elseif q==1    
    %When plant is in T1 ("Rod One")
    if control ==remove1
        qNext=0;
        reset=1;
    else
        qNext=1;
        reset=0;
    end;

elseif q==2    
    %When plant is in T2 ("Rod Two")
    if control ==remove2
        qNext=0;
        reset=1;
    else
        qNext=2;
        reset=0;
    end;
else
    qNext=-1; %this should never execute
    reset=-1; %this should never execute
end

== matlab function nuclearReactor/Plant14/MATLAB Function1 ==
  data: x input; x_dot0 output; x_dot1 output; x_dot2 output
function [x_dot0, x_dot1, x_dot2] = ODEs(x)
%#codegen
x_dot0=0.1*x-50;
x_dot1=0.1*x-56;
x_dot2=0.1*x-60;

== matlab function nuclearReactor/Controller15/MATLAB Function ==
  data: q input; qNext output; x input; r1 output; r2 output; y1 input; y2 input; control output


function [qNext,r1,r2,control]  = phi(q, x, y1, y2)
%#codegen
% control {-1 undefined, 0 add1, 1 remove1, 2 add2, 3 remove2}

undef =0;
add1 = 1;
remove1 =2;
add2 = 3;
remove2 =4;
c=15;

if q==0 
    %When plant is in T0 ("No Rod")
    if x > 550 && y1 >= c && y2<c
        qNext=1;
        r1=0; r2=0;
        control=add1;
    elseif x>550 && y2>=c
        qNext=2;
        r1=0; r2=0;
        control=add2;
    else
        qNext=0;
        r1=0; r2=0;
        control=undef;
    end;
    
elseif q==1    
    %When plant is in T1 ("Rod One")
    if x <= 510 
        qNext=0;
        r1=1; r2=0;
        control=remove1;
    else
        qNext=1;
        r1=0; r2=0;
        control=undef;
    end;

elseif q==2    
    %When plant is in T2 ("Rod Two")
    if x <= 510 
        qNext=0;
        r1=0; r2=1;
        control=remove2;
    else
        qNext=2;
        r1=0; r2=0;
        control=undef;
    end;
else
    qNext=-1; %this should never execute
    r1=0; r2=0; %this should never execute
    control=-1; %this should never execute
end

== matlab function nuclearReactor/Controller16/MATLAB Function ==
  data: q input; qNext output; x input; r1 output; r2 output; y1 input; y2 input; control output


function [qNext,r1,r2,control]  = phi(q, x, y1, y2)
%#codegen
% control {-1 undefined, 0 add1, 1 remove1, 2 add2, 3 remove2}

undef =0;
add1 = 1;
remove1 =2;
add2 = 3;
remove2 =4;
c=15;

if q==0 
    %When plant is in T0 ("No Rod")
    if x > 550 && y1 >= c && y2<c
        qNext=1;
        r1=0; r2=0;
        control=add1;
    elseif x>550 && y2>=c
        qNext=2;
        r1=0; r2=0;
        control=add2;
    else
        qNext=0;
        r1=0; r2=0;
        control=undef;
    end;
    
elseif q==1    
    %When plant is in T1 ("Rod One")
    if x <= 510 
        qNext=0;
        r1=1; r2=0;
        control=remove1;
    else
        qNext=1;
        r1=0; r2=0;
        control=undef;
    end;

elseif q==2    
    %When plant is in T2 ("Rod Two")
    if x <= 510 
        qNext=0;
        r1=0; r2=1;
        control=remove2;
    else
        qNext=2;
        r1=0; r2=0;
        control=undef;
    end;
else
    qNext=-1; %this should never execute
    r1=0; r2=0; %this should never execute
    control=-1; %this should never execute
end

== matlab function nuclearReactor/Controller17/MATLAB Function ==
  data: q input; qNext output; x input; r1 output; r2 output; y1 input; y2 input; control output


function [qNext,r1,r2,control]  = phi(q, x, y1, y2)
%#codegen
% control {-1 undefined, 0 add1, 1 remove1, 2 add2, 3 remove2}

undef =0;
add1 = 1;
remove1 =2;
add2 = 3;
remove2 =4;
c=15;

if q==0 
    %When plant is in T0 ("No Rod")
    if x > 550 && y1 >= c && y2<c
        qNext=1;
        r1=0; r2=0;
        control=add1;
    elseif x>550 && y2>=c
        qNext=2;
        r1=0; r2=0;
        control=add2;
    else
        qNext=0;
        r1=0; r2=0;
        control=undef;
    end;
    
elseif q==1    
    %When plant is in T1 ("Rod One")
    if x <= 510 
        qNext=0;
        r1=1; r2=0;
        control=remove1;
    else
        qNext=1;
        r1=0; r2=0;
        control=undef;
    end;

elseif q==2    
    %When plant is in T2 ("Rod Two")
    if x <= 510 
        qNext=0;
        r1=0; r2=1;
        control=remove2;
    else
        qNext=2;
        r1=0; r2=0;
        control=undef;
    end;
else
    qNext=-1; %this should never execute
    r1=0; r2=0; %this should never execute
    control=-1; %this should never execute
end

== matlab function nuclearReactor/Controller18/MATLAB Function ==
  data: q input; qNext output; x input; r1 output; r2 output; y1 input; y2 input; control output


function [qNext,r1,r2,control]  = phi(q, x, y1, y2)
%#codegen
% control {-1 undefined, 0 add1, 1 remove1, 2 add2, 3 remove2}

undef =0;
add1 = 1;
remove1 =2;
add2 = 3;
remove2 =4;
c=15;

if q==0 
    %When plant is in T0 ("No Rod")
    if x > 550 && y1 >= c && y2<c
        qNext=1;
        r1=0; r2=0;
        control=add1;
    elseif x>550 && y2>=c
        qNext=2;
        r1=0; r2=0;
        control=add2;
    else
        qNext=0;
        r1=0; r2=0;
        control=undef;
    end;
    
elseif q==1    
    %When plant is in T1 ("Rod One")
    if x <= 510 
        qNext=0;
        r1=1; r2=0;
        control=remove1;
    else
        qNext=1;
        r1=0; r2=0;
        control=undef;
    end;

elseif q==2    
    %When plant is in T2 ("Rod Two")
    if x <= 510 
        qNext=0;
        r1=0; r2=1;
        control=remove2;
    else
        qNext=2;
        r1=0; r2=0;
        control=undef;
    end;
else
    qNext=-1; %this should never execute
    r1=0; r2=0; %this should never execute
    control=-1; %this should never execute
end

== matlab function nuclearReactor/Controller19/MATLAB Function ==
  data: q input; qNext output; x input; r1 output; r2 output; y1 input; y2 input; control output


function [qNext,r1,r2,control]  = phi(q, x, y1, y2)
%#codegen
% control {-1 undefined, 0 add1, 1 remove1, 2 add2, 3 remove2}

undef =0;
add1 = 1;
remove1 =2;
add2 = 3;
remove2 =4;
c=15;

if q==0 
    %When plant is in T0 ("No Rod")
    if x > 550 && y1 >= c && y2<c
        qNext=1;
        r1=0; r2=0;
        control=add1;
    elseif x>550 && y2>=c
        qNext=2;
        r1=0; r2=0;
        control=add2;
    else
        qNext=0;
        r1=0; r2=0;
        control=undef;
    end;
    
elseif q==1    
    %When plant is in T1 ("Rod One")
    if x <= 510 
        qNext=0;
        r1=1; r2=0;
        control=remove1;
    else
        qNext=1;
        r1=0; r2=0;
        control=undef;
    end;

elseif q==2    
    %When plant is in T2 ("Rod Two")
    if x <= 510 
        qNext=0;
        r1=0; r2=1;
        control=remove2;
    else
        qNext=2;
        r1=0; r2=0;
        control=undef;
    end;
else
    qNext=-1; %this should never execute
    r1=0; r2=0; %this should never execute
    control=-1; %this should never execute
end
